simulink model "vibration_data_operation_sm"  (R2017a)
settings: Solver=VariableStepAuto  StartTime=0.0  StopTime=120  RelTol=1e-3
settings Model: Creator=Chaohua Zhao  LastModifiedBy=Chaohua Zhao

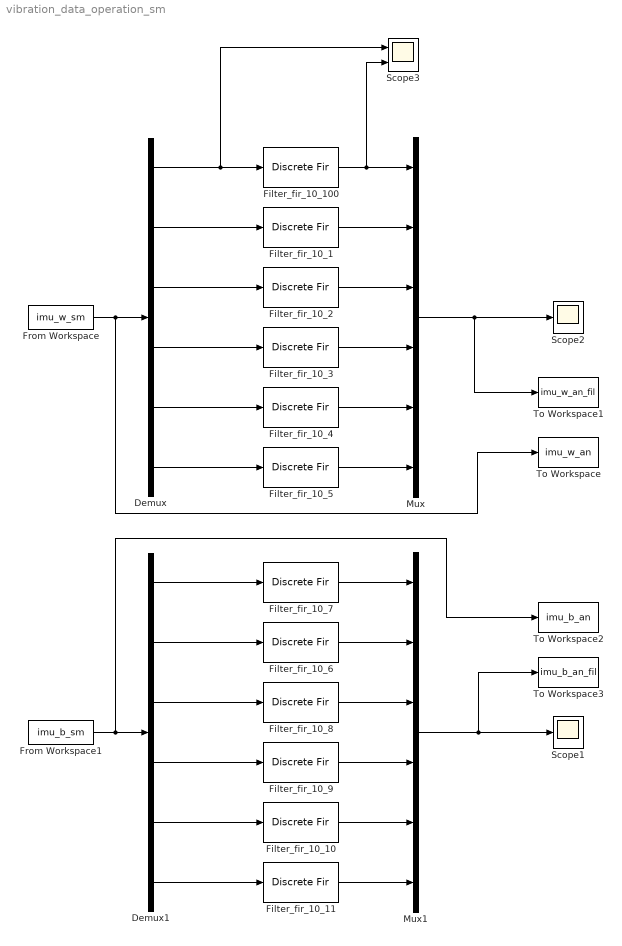
== system vibration_data_operation_sm ==
  Demux : Demux  Outputs=6
  Demux1 : Demux  Outputs=6
  Filter_fir_10_{1..11,100} (12 alike) : DiscreteFir  Tag=BlockMethodSubSystem  Coefficients=[0 0.0054786758595111026 0.042763636162144819 0.12151889269739169 0.20757905037865335 0.245319489804598 0.20757905037865335 0.12151889269739169 0.042763636162144819 0.0054786758595111026 0]  InputProcessing=Columns as channels (frame based)
  From Workspace : FromWorkspace  VariableName=imu_w_sm  SampleTime=0.003  OutputAfterFinalValue=Setting to zero
  From Workspace1 : FromWorkspace  VariableName=imu_b_sm  SampleTime=0.003  OutputAfterFinalValue=Setting to zero
  Mux : Mux  Inputs=6
  Mux1 : Mux  Inputs=6
  Scope1 : Scope
  Scope2 : Scope
  Scope3 : Scope  NumInputPorts=2
  To Workspace : ToWorkspace  VariableName=imu_w_an  SampleTime=-1
  To Workspace1 : ToWorkspace  VariableName=imu_w_an_fil  SampleTime=-1
  To Workspace2 : ToWorkspace  VariableName=imu_b_an  SampleTime=-1
  To Workspace3 : ToWorkspace  VariableName=imu_b_an_fil  SampleTime=-1
  wires:
  From Workspace/1 -> To Workspace/1, Demux/1
  Demux/1 -> Scope3/1, Filter_fir_10_100/1
  Demux/2 -> Filter_fir_10_1/1
  Demux/6 -> Filter_fir_10_5/1
  Demux/5 -> Filter_fir_10_4/1
  Demux/4 -> Filter_fir_10_3/1
  Demux/3 -> Filter_fir_10_2/1
  Filter_fir_10_100/1 -> Scope3/2, Mux/1
  Filter_fir_10_1/1 -> Mux/2
  Filter_fir_10_3/1 -> Mux/4
  Filter_fir_10_4/1 -> Mux/5
  Filter_fir_10_5/1 -> Mux/6
  Filter_fir_10_2/1 -> Mux/3
  Mux/1 -> To Workspace1/1, Scope2/1
  Mux1/1 -> To Workspace3/1, Scope1/1
  Filter_fir_10_8/1 -> Mux1/3
  Filter_fir_10_11/1 -> Mux1/6
  Filter_fir_10_10/1 -> Mux1/5
  Filter_fir_10_9/1 -> Mux1/4
  Filter_fir_10_6/1 -> Mux1/2
  Filter_fir_10_7/1 -> Mux1/1
  Demux1/3 -> Filter_fir_10_8/1
  Demux1/4 -> Filter_fir_10_9/1
  Demux1/5 -> Filter_fir_10_10/1
  Demux1/6 -> Filter_fir_10_11/1
  Demux1/2 -> Filter_fir_10_6/1
  Demux1/1 -> Filter_fir_10_7/1
  From Workspace1/1 -> To Workspace2/1, Demux1/1
